simulink model "HandOn_SSD_3"  (R2023b)
settings: Solver=VariableStepAuto  StartTime=0.0  StopTime=T_stop  RelTol=1e-3
undefined symbols (not defined in the file): x_0
settings Model: Creator=lloss  LastModifiedBy=lloss
settings DataIOCC: SaveFormat=Array

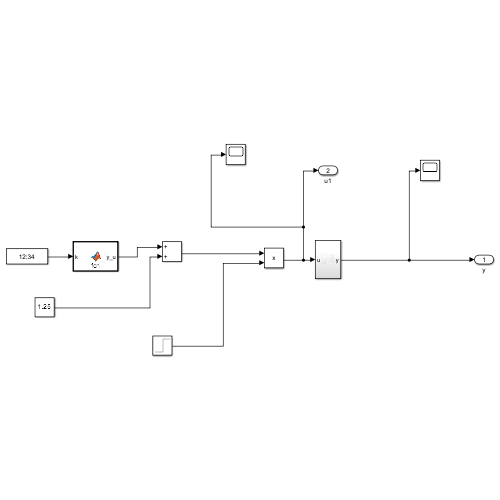
[thumbnail: Simulink's stored preview of the top-level diagram]
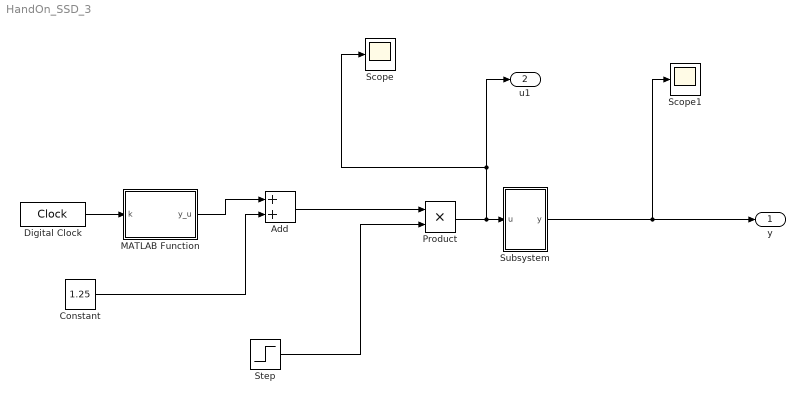
== system HandOn_SSD_3 ==
  Add : Sum
  Constant : Constant  Value=1.25
  Digital Clock : DigitalClock
  MATLAB Function : MATLAB Function  TreatAsAtomicUnit=on
  Product : Product
  Scope : Scope
  Scope1 : Scope
  Step : Step  Time=0  SampleTime=1
  Subsystem : Subsystem
  y : Outport
  u1 : Outport  Port=2
  wires:
  Subsystem/1(y) -> Scope1/1, y/1
  Digital Clock/1 -> MATLAB Function/1(k)
  Add/1 -> Product/1
  MATLAB Function/1(y_u) -> Add/1
  Constant/1 -> Add/2
  Step/1 -> Product/2
  Product/1 -> Scope/1, u1/1, Subsystem/1(u)

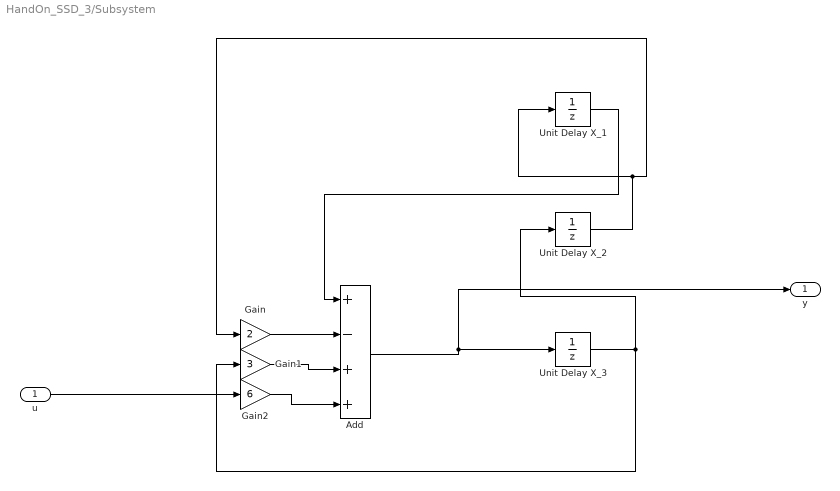
== system HandOn_SSD_3/Subsystem ==
  u : Inport
  Add : Sum  Inputs=+-++
  Gain : Gain  Gain=2
  Gain1 : Gain  Gain=3
  Gain2 : Gain  Gain=6
  Unit Delay X_1 : UnitDelay  InitialCondition=x_0(1)  SampleTime=-1  HasFrameUpgradeWarning=on
  Unit Delay X_2 : UnitDelay  InitialCondition=x_0(2)  SampleTime=-1  HasFrameUpgradeWarning=on
  Unit Delay X_3 : UnitDelay  InitialCondition=x_0(3)  SampleTime=-1  HasFrameUpgradeWarning=on
  y : Outport
  wires:
  Gain/1 -> Add/2
  u/1 -> Gain2/1
  Add/1 -> y/1, Unit Delay X_3/1
  Gain2/1 -> Add/4
  Unit Delay X_3/1 -> Unit Delay X_2/1, Gain1/1
  Unit Delay X_2/1 -> Unit Delay X_1/1, Gain/1
  Gain1/1 -> Add/3
  Unit Delay X_1/1 -> Add/1

== matlab function HandOn_SSD_3/MATLAB Function ==
  data: k input; y_u output
function y_u = fcn(k)
y_u = -(2/3)^k;
